simulink model "ejemplo_simulink"  (R2016a)
settings: Solver=FixedStepDiscrete  StartTime=0.0  StopTime=inf  FixedStep=0.001  RelTol=1e-3
libraries: LibrarySimulinkSAS x1, aerolibanimutils x1
settings Model: Creator=PC  LastModifiedBy=PC

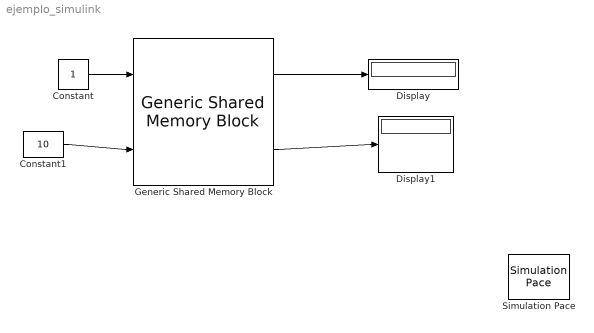
== system ejemplo_simulink ==
  Constant : Constant  OutDataTypeStr=single  SampleTime=-1
  Constant1 : Constant  Value=10  OutDataTypeStr=single
  Display : Display
  Display1 : Display
  Generic Shared Memory Block : LibrarySimulinkSAS/Generic Shared Memory Block  nombre='ARDUINO'  dispositivo=1  vecE=[1 1]  vecS=[1 1]  tipoE=['f' 'f']  tipoS=['f' 'f']  ts=-1
  Simulation Pace : aerolibanimutils/Simulation Pace  SimulationPace=1  SleepMode=MATLAB Thread  OutputPaceError=off  SampleTime=-1
  wires:
  Constant/1 -> Generic Shared Memory Block/1
  Generic Shared Memory Block/1 -> Display/1
  Generic Shared Memory Block/2 -> Display1/1
  Constant1/1 -> Generic Shared Memory Block/2
